simulink model "dyskretyzacja1"  (R2018a)
settings: Solver=FixedStepDiscrete  StartTime=0.0  StopTime=10.0  FixedStep=T  RelTol=1e-3
undefined symbols (not defined in the file or in its folder): T
settings Model: Creator=Dominik  LastModifiedBy=Dominik

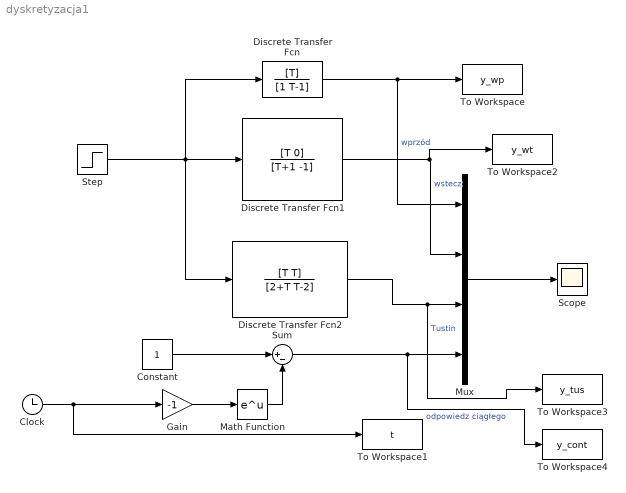
== system dyskretyzacja1 ==
  Clock : Clock
  Constant : Constant
  Discrete Transfer Fcn : DiscreteTransferFcn  Numerator=[T]  Denominator=[1 T-1]  SampleTime=T
  Discrete Transfer Fcn1 : DiscreteTransferFcn  Numerator=[T 0]  Denominator=[T+1 -1]  SampleTime=T
  Discrete Transfer Fcn2 : DiscreteTransferFcn  Numerator=[T T]  Denominator=[2+T T-2]  SampleTime=T
  Gain : Gain  Gain=-1
  Math Function : Math  SaturateOnIntegerOverflow=on
  Mux : Mux
  Scope : Scope
  Step : Step  Time=0  SampleTime=0
  Sum : Sum  Inputs=|+-
  To Workspace : ToWorkspace  VariableName=y_wp  SampleTime=-1
  To Workspace1 : ToWorkspace  VariableName=t  SampleTime=-1
  To Workspace2 : ToWorkspace  VariableName=y_wt  SampleTime=-1
  To Workspace3 : ToWorkspace  VariableName=y_tus  SampleTime=-1
  To Workspace4 : ToWorkspace  VariableName=y_cont  SampleTime=-1
  wires:
  Gain/1 -> Math Function/1
  Clock/1 -> To Workspace1/1, Gain/1
  Constant/1 -> Sum/1
  Math Function/1 -> Sum/2
  Step/1 -> Discrete Transfer Fcn/1, Discrete Transfer Fcn1/1, Discrete Transfer Fcn2/1
  Sum/1 -> To Workspace4/1, Mux/4  "odpowiedz ciągłego"
  Discrete Transfer Fcn/1 -> To Workspace/1, Mux/1  "wprzód"
  Discrete Transfer Fcn2/1 -> To Workspace3/1, Mux/3  "Tustin"
  Discrete Transfer Fcn1/1 -> To Workspace2/1, Mux/2  "wstecz"
  Mux/1 -> Scope/1
